simulink model "Practica1simulink"  (R2025a)
settings: Solver=VariableStepAuto  StartTime=0.0  StopTime=10.0  RelTol=1e-3
undefined symbols (not defined in the file): Beq, Bp, Fc, g, Ip, Lp, Mc, Mp
settings Model: LastModifiedBy=Francisco

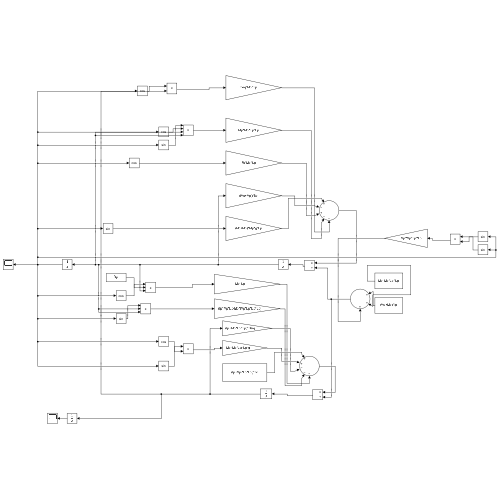
[thumbnail: Simulink's stored preview of the top-level diagram]
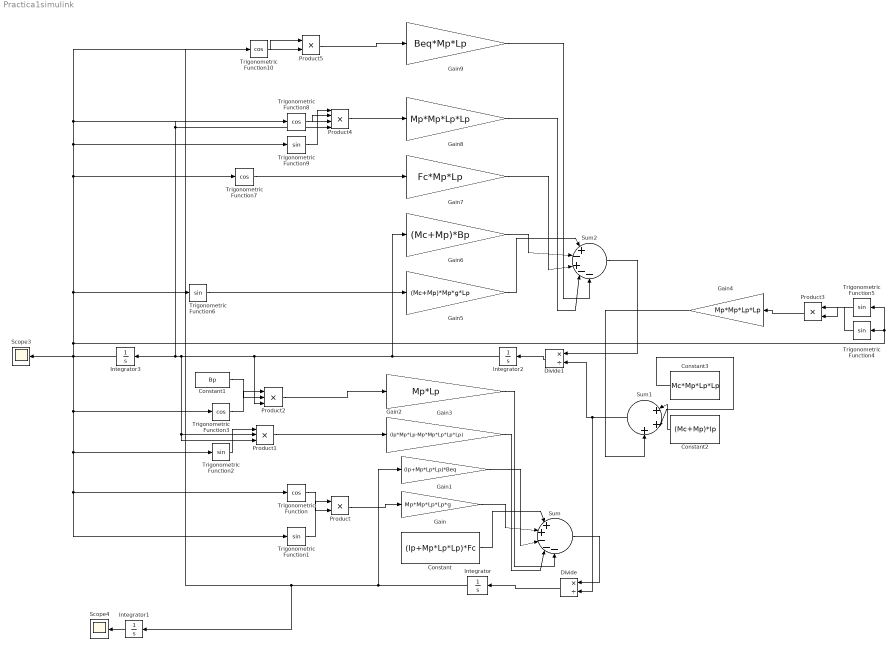
== system Practica1simulink ==
  Constant : Constant  Value=(Ip+Mp*Lp*Lp)*Fc
  Constant1 : Constant  Value=Bp
  Constant2 : Constant  Value=(Mc+Mp)*Ip
  Constant3 : Constant  Value=Mc*Mp*Lp*Lp
  Divide : Product  Inputs=*/
  Divide1 : Product  Inputs=*/
  Gain : Gain  Gain=Mp*Mp*Lp*Lp*g
  Gain1 : Gain  Gain=(Ip+Mp*Lp*Lp)*Beq
  Gain2 : Gain  Gain=(Ip*Mp*Lp-Mp*Mp*Lp*Lp*Lp)
  Gain3 : Gain  Gain=Mp*Lp
  Gain4 : Gain  Gain=Mp*Mp*Lp*Lp
  Gain5 : Gain  Gain=(Mc+Mp)*Mp*g*Lp
  Gain6 : Gain  Gain=(Mc+Mp)*Bp
  Gain7 : Gain  Gain=Fc*Mp*Lp
  Gain8 : Gain  Gain=Mp*Mp*Lp*Lp
  Gain9 : Gain  Gain=Beq*Mp*Lp
  Integrator : Integrator
  Integrator1 : Integrator
  Integrator2 : Integrator
  Integrator3 : Integrator  InitialCondition=pi/180
  Product : Product
  Product1 : Product  Inputs=3
  Product2 : Product  Inputs=3
  Product3 : Product
  Product4 : Product  Inputs=4
  Product5 : Product
  Scope3 : Scope
      settings: ActiveDisplayYMinimum=-12.296569831701518  ActiveDisplayYMaximum=110.84366141051312  DataLoggingVariableName=ScopeData3
  Scope4 : Scope
      settings: ActiveDisplayYMinimum=-0.019299274218518649  ActiveDisplayYMaximum=0.17369346796666787  DataLoggingVariableName=ScopeData4
  Sum : Sum  Inputs=|++---
  Sum1 : Sum  Inputs=|+++
  Sum2 : Sum  Inputs=|+-+--
  Trigonometric Function{,3,7..8,10} (5 alike) : Trigonometry  Operator=cos
  Trigonometric Function{1..2,4..6,9} (6 alike) : Trigonometry
  wires:
  Constant/1 -> Sum/1
  Gain/1 -> Sum/2
  Product/1 -> Gain/1
  Trigonometric Function/1 -> Product/2
  Trigonometric Function1/1 -> Product/1
  Gain1/1 -> Sum/3
  Product1/1 -> Gain2/1
  Trigonometric Function2/1 -> Product1/1
  Integrator3/1 -> Trigonometric Function1/1, Trigonometric Function/1, Trigonometric Function2/1, Trigonometric Function3/1, Trigonometric Function5/1, Trigonometric Function4/1, Trigonometric Function10/1, Trigonometric Function8/1, Trigonometric Function9/1, Trigonometric Function7/1, Trigonometric Function6/1, Scope3/1
  Integrator1/1 -> Scope4/1
  Gain2/1 -> Sum/4
  Trigonometric Function3/1 -> Product2/1
  Constant1/1 -> Product2/2
  Product2/1 -> Gain3/1
  Gain3/1 -> Sum/5
  Divide/1 -> Integrator/1
  Product3/1 -> Gain4/1
  Trigonometric Function5/1 -> Product3/2
  Trigonometric Function4/1 -> Product3/1
  Gain4/1 -> Sum1/3
  Constant3/1 -> Sum1/2
  Constant2/1 -> Sum1/1
  Sum/1 -> Divide/1
  Trigonometric Function6/1 -> Gain5/1
  Gain5/1 -> Sum2/1
  Gain6/1 -> Sum2/2
  Trigonometric Function7/1 -> Gain7/1
  Gain7/1 -> Sum2/3
  Trigonometric Function9/1 -> Product4/1
  Trigonometric Function8/1 -> Product4/2
  Product4/1 -> Gain8/1
  Gain8/1 -> Sum2/4
  Product5/1 -> Gain9/1
  Trigonometric Function10/1 -> Product5/1
  Gain9/1 -> Sum2/5
  Sum2/1 -> Divide1/1
  Sum1/1 -> Divide/2, Divide1/2
  Divide1/1 -> Integrator2/1
  Integrator/1 -> Product5/2, Integrator1/1, Gain1/1
  Integrator2/1 -> Product1/3, Product1/2, Product4/3, Product4/4, Integrator3/1, Product2/3, Gain6/1
